simulink model "Laser_Knight_Team9"  (R2019a)
settings: Solver=VariableStepAuto  StartTime=0.0  StopTime=10.0  RelTol=1e-3
libraries: arduinolib x34
settings Model: Creator=user  LastModifiedBy=user

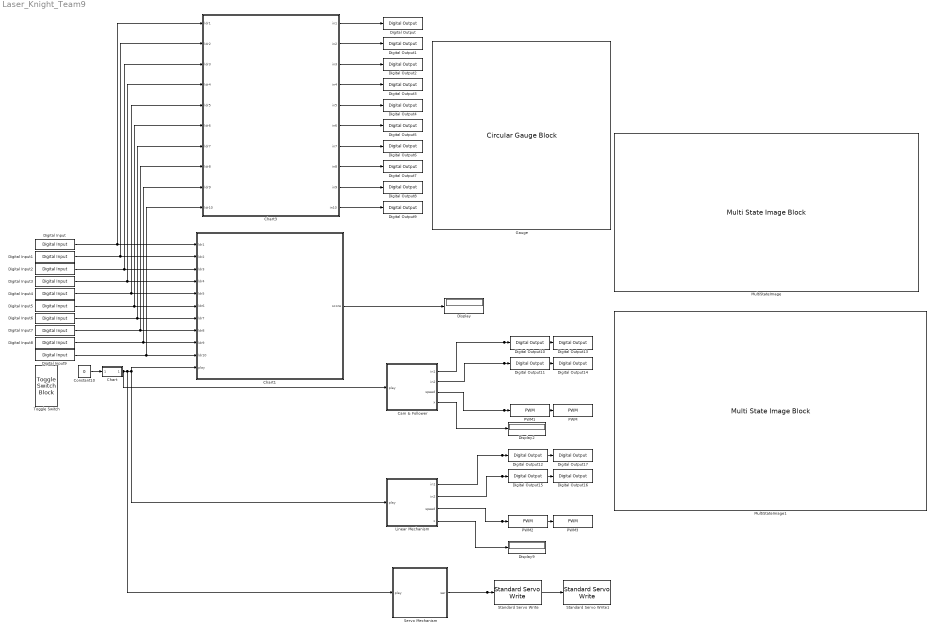
== system Laser_Knight_Team9 ==
  Cam & Follower : Stateflow chart  BlockKeywords=__PRM__SERIALIZED__DATA__:Stateflow Chart,Stateflow Diagram  TreatAsAtomicUnit=on
  Chart : Stateflow chart  BlockKeywords=__PRM__SERIALIZED__DATA__:Stateflow Chart,Stateflow Diagram  TreatAsAtomicUnit=on
  Chart1 : Stateflow chart  BlockKeywords=__PRM__SERIALIZED__DATA__:Stateflow Chart,Stateflow Diagram  TreatAsAtomicUnit=on
  Chart3 : Stateflow chart  BlockKeywords=__PRM__SERIALIZED__DATA__:Stateflow Chart,Stateflow Diagram  TreatAsAtomicUnit=on
  Constant10 : Constant  Value=0
  Digital Input : arduinolib/Digital Input  pinNumber=22  sampleTime=0.001  blockPlatform=arduino
      settings: SourceProductName=Simulink Support Package for Arduino Hardware
  Digital Input1 : arduinolib/Digital Input  pinNumber=24  sampleTime=0.1  blockPlatform=arduino
      settings: SourceProductName=Simulink Support Package for Arduino Hardware
  Digital Input2 : arduinolib/Digital Input  pinNumber=26  sampleTime=0.1  blockPlatform=arduino
      settings: SourceProductName=Simulink Support Package for Arduino Hardware
  Digital Input3 : arduinolib/Digital Input  pinNumber=28  sampleTime=0.1  blockPlatform=arduino
      settings: SourceProductName=Simulink Support Package for Arduino Hardware
  Digital Input4 : arduinolib/Digital Input  pinNumber=30  sampleTime=0.1  blockPlatform=arduino
      settings: SourceProductName=Simulink Support Package for Arduino Hardware
  Digital Input5 : arduinolib/Digital Input  pinNumber=32  sampleTime=0.1  blockPlatform=arduino
      settings: SourceProductName=Simulink Support Package for Arduino Hardware
  Digital Input6 : arduinolib/Digital Input  pinNumber=34  sampleTime=0.1  blockPlatform=arduino
      settings: SourceProductName=Simulink Support Package for Arduino Hardware
  Digital Input7 : arduinolib/Digital Input  pinNumber=36  sampleTime=0.1  blockPlatform=arduino
      settings: SourceProductName=Simulink Support Package for Arduino Hardware
  Digital Input8 : arduinolib/Digital Input  pinNumber=38  sampleTime=0.1  blockPlatform=arduino
      settings: SourceProductName=Simulink Support Package for Arduino Hardware
  Digital Input9 : arduinolib/Digital Input  pinNumber=40  sampleTime=0.1  blockPlatform=arduino
      settings: SourceProductName=Simulink Support Package for Arduino Hardware
  Digital Output : arduinolib/Digital Output  pinNumber=42  blockPlatform=arduino
  Digital Output1 : arduinolib/Digital Output  pinNumber=44  blockPlatform=arduino
  Digital Output10 : arduinolib/Digital Output  pinNumber=8  blockPlatform=arduino
  Digital Output11 : arduinolib/Digital Output  pinNumber=10  blockPlatform=arduino
  Digital Output12 : arduinolib/Digital Output  pinNumber=12  blockPlatform=arduino
  Digital Output13 : arduinolib/Digital Output  pinNumber=9  blockPlatform=arduino
  Digital Output14 : arduinolib/Digital Output  pinNumber=11  blockPlatform=arduino
  Digital Output15 : arduinolib/Digital Output  pinNumber=14  blockPlatform=arduino
  Digital Output16 : arduinolib/Digital Output  pinNumber=15  blockPlatform=arduino
  Digital Output17 : arduinolib/Digital Output  pinNumber=13  blockPlatform=arduino
  Digital Output2 : arduinolib/Digital Output  pinNumber=46  blockPlatform=arduino
  Digital Output3 : arduinolib/Digital Output  pinNumber=48  blockPlatform=arduino
  Digital Output4 : arduinolib/Digital Output  pinNumber=50  blockPlatform=arduino
  Digital Output5 : arduinolib/Digital Output  pinNumber=52  blockPlatform=arduino
  Digital Output6 : arduinolib/Digital Output  pinNumber=37  blockPlatform=arduino
  Digital Output7 : arduinolib/Digital Output  pinNumber=39  blockPlatform=arduino
  Digital Output8 : arduinolib/Digital Output  pinNumber=41  blockPlatform=arduino
  Digital Output9 : arduinolib/Digital Output  pinNumber=43  blockPlatform=arduino
  Display : Display
  Display2 : Display
  Display9 : Display
  Gauge : CircularGaugeBlock  LabelPosition=Hide  ScaleMax=300  TickInterval=20
  Linear Mechanism : Stateflow chart  BlockKeywords=__PRM__SERIALIZED__DATA__:Stateflow Chart,Stateflow Diagram  TreatAsAtomicUnit=on
  MultiStateImage : MultiStateImageBlock  LabelPosition=Hide  ScaleMode=Fill
  MultiStateImage1 : MultiStateImageBlock  LabelPosition=Hide  ScaleMode=Fill
  PWM : arduinolib/PWM  pinNumber=4  EnableInputFrequency=off  InitialFrequency=2000  InitialDutyCycle=0  NotificationType=None  blockPlatform=arduino
  PWM1 : arduinolib/PWM  pinNumber=5  EnableInputFrequency=off  InitialFrequency=2000  InitialDutyCycle=0  NotificationType=None  blockPlatform=arduino
  PWM2 : arduinolib/PWM  pinNumber=6  EnableInputFrequency=off  InitialFrequency=2000  InitialDutyCycle=0  NotificationType=None  blockPlatform=arduino
  PWM3 : arduinolib/PWM  pinNumber=7  EnableInputFrequency=off  InitialFrequency=2000  InitialDutyCycle=0  NotificationType=None  blockPlatform=arduino
  Servo Mechanism : Stateflow chart  BlockKeywords=__PRM__SERIALIZED__DATA__:Stateflow Chart,Stateflow Diagram  TreatAsAtomicUnit=on
  Standard Servo Write : arduinolib/Standard Servo Write  pinNumber=31  ServoIndex=0  blockPlatform=ARDUINO
      settings: SourceProductName=Simulink Support Package for Arduino Hardware
  Standard Servo Write1 : arduinolib/Standard Servo Write  pinNumber=33  ServoIndex=0  blockPlatform=ARDUINO
      settings: SourceProductName=Simulink Support Package for Arduino Hardware
  Toggle Switch : ToggleSwitchBlock  LabelPosition=Hide
      settings: Values={{'Off', 'On'}, [0 1]}
  wires:
  Chart3/5(in5) -> Digital Output4/1
  Linear Mechanism/4(x) -> Display9/1
  Chart3/8(in8) -> Digital Output7/1
  Servo Mechanism/1(ser) -> Standard Servo Write1/1, Standard Servo Write/1
  Chart3/3(in3) -> Digital Output2/1
  Cam & Follower/4(x) -> Display2/1
  Cam & Follower/1(in1) -> Digital Output13/1, Digital Output10/1
  Cam & Follower/3(speed) -> PWM/1, PWM1/1
  Cam & Follower/2(in2) -> Digital Output14/1, Digital Output11/1
  Digital Input6/1 -> Chart3/7(ldr7), Chart1/7(ldr7)
  Digital Input4/1 -> Chart3/5(ldr5), Chart1/5(ldr5)
  Digital Input2/1 -> Chart3/3(ldr3), Chart1/3(ldr3)
  Digital Input5/1 -> Chart3/6(ldr6), Chart1/6(ldr6)
  Digital Input/1 -> Chart3/1(ldr1), Chart1/1(ldr1)
  Digital Input7/1 -> Chart3/8(ldr8), Chart1/8(ldr8)
  Linear Mechanism/3(speed) -> PWM3/1, PWM2/1
  Digital Input9/1 -> Chart3/10(ldr10), Chart1/10(ldr10)
  Digital Input8/1 -> Chart3/9(ldr9), Chart1/9(ldr9)
  Chart/1(play) -> Cam & Follower/1(play), Servo Mechanism/1(play), Linear Mechanism/1(play), Chart1/11(play)
  Linear Mechanism/2(in2) -> Digital Output16/1, Digital Output15/1
  Digital Input3/1 -> Chart3/4(ldr4), Chart1/4(ldr4)
  Chart3/4(in4) -> Digital Output3/1
  Chart3/1(in1) -> Digital Output/1
  Chart1/1(score) -> Display/1
  Digital Input1/1 -> Chart3/2(ldr2), Chart1/2(ldr2)
  Chart3/10(in10) -> Digital Output9/1
  Chart3/2(in2) -> Digital Output1/1
  Chart3/6(in6) -> Digital Output5/1
  Chart3/7(in7) -> Digital Output6/1
  Constant10/1 -> Chart/1(game)
  Chart3/9(in9) -> Digital Output8/1
  Linear Mechanism/1(in1) -> Digital Output17/1, Digital Output12/1

== stateflow chart Laser_Knight_Team9/Chart1 ==
  state Gameplay
    state initial
      score=0;
    state Score
      state LDR1 [parallel]
        settings: executionOrder=1
        state Score1
          score=score;
        state LDR1
          score=score;
        (default) -> Gameplay.Score.LDR1.Score1
        Gameplay.Score.LDR1.Score1 -> Gameplay.Score.LDR1.LDR1 : [ldr1==0||ldr2==0]{score=score+10;}
        Gameplay.Score.LDR1.LDR1 -> Gameplay.Score.LDR1.Score1 : [after(3,sec)]
      state LDR2 [parallel]
        settings: executionOrder=2
        state Score1
          score=score;
        state LDR1
          score=score;
        (default) -> Gameplay.Score.LDR2.Score1
        Gameplay.Score.LDR2.Score1 -> Gameplay.Score.LDR2.LDR1 : [ldr3==0||ldr4==0]{score=score+20}
        Gameplay.Score.LDR2.LDR1 -> Gameplay.Score.LDR2.Score1 : [after(3,sec)]
      state LDR3 [parallel]
        settings: executionOrder=3
        state Score1
          score=score;
        state LDR1
          score=score;
        (default) -> Gameplay.Score.LDR3.Score1
        Gameplay.Score.LDR3.Score1 -> Gameplay.Score.LDR3.LDR1 : [ldr5==0||ldr6==0]{score=score+30}
        Gameplay.Score.LDR3.LDR1 -> Gameplay.Score.LDR3.Score1 : [after(3,sec)]
      state LDR4 [parallel]
        settings: executionOrder=4
        state Score1
          score=score;
        state LDR1
          score=score;
        (default) -> Gameplay.Score.LDR4.Score1
        Gameplay.Score.LDR4.Score1 -> Gameplay.Score.LDR4.LDR1 : [ldr7==0||ldr8==0]{score=score+40}
        Gameplay.Score.LDR4.LDR1 -> Gameplay.Score.LDR4.Score1 : [after(3,sec)]
      state LDR5 [parallel]
        settings: executionOrder=5
        state Score1
          score=score;
        state LDR1
          score=score;
        (default) -> Gameplay.Score.LDR5.Score1
        Gameplay.Score.LDR5.Score1 -> Gameplay.Score.LDR5.LDR1 : [ldr9==0||ldr10==0]{score=score+50}
        Gameplay.Score.LDR5.LDR1 -> Gameplay.Score.LDR5.Score1 : [after(3,sec)]
    (default) -> initial
    initial -> Score
  state GameOver
    score=score;
  (default) -> Gameplay
  Gameplay -> GameOver : [play==0]
  GameOver -> Gameplay : [play==1]
  data: score output; ldr1 input; ldr2 input; ldr3 input; ldr4 input; ldr5 input; ldr6 input; ldr7 input; ldr8 input; ldr9 input; ldr10 input; play input

== stateflow chart Laser_Knight_Team9/Servo Mechanism ==
  state move1
    ser=ser;
  state initial
    ser=10
  state move2
    ser=ser;
  move1 -> move1 [order 2] : [after(50,msec)&&ser<170]{ser = ser + 1}
  (default) -> initial
  initial -> move1 : [play==1]
  move1 -> move2 [order 1] : [ser==170]
  move2 -> move1 [order 1] : [ser==10]
  move2 -> initial [order 3] : [play==0]
  move2 -> move2 [order 2] : [after(50,msec)&&ser>10]{ser = ser - 1}
  data: ser output; play input

== stateflow chart Laser_Knight_Team9/Cam & Follower ==
  state Gameplay
    x=2;
    state Initial
      speed=200;
      in1=0;
      in2=0;
    state Final
      state Motor2
        speed=speed
        in1=1
        in2=0
        x=0
      state Motor1
        speed=speed
        in1=0
        in2=1
        x=0
      (default) -> Motor1
      Motor2 -> Motor1 : [after(10,sec)]{speed=speed+5}
      Motor1 -> Motor2 : [after(10,sec)]{speed=speed+5}
    (default) -> Initial
    Initial -> Final : [speed==200 && play==1]
    Final -> Initial : [speed>=255]
  state GameOver
    x=1;
    in1=0;
    in2=0;
    speed=200;
  (default) -> Gameplay
  Gameplay -> GameOver : [play==0]
  GameOver -> Gameplay : [x==1&&play==1]
  data: in1 output; in2 output; speed output; x output =0; play input

== stateflow chart Laser_Knight_Team9/Chart ==
  state Time
    t=180;
    state Time1
      t=t;
      play=1;
    state Time2
      t=t;
      play=1;
    Time1 -> Time2 : [after(1,sec)&&game==1]{t = t - 1}
    (default) -> Time1
    Time2 -> Time1 : [after(1,sec)&&game==1]{t = t - 1}
  state GameOver
    play=0;
  (default) -> Time
  Time -> GameOver : [t==0 || game==0]
  GameOver -> Time : [game==1]
  data: play output =1; t local =180; game input

== stateflow chart Laser_Knight_Team9/Linear Mechanism ==
  state Gameplay
    state Final
      state Motor2
        speed=255
        in1=1
        in2=0
        x=0
      state Motor1
        speed=255
        in1=0
        in2=1
        x=0
      (default) -> Motor1
      Motor2 -> Motor1 : [after(8,sec)&&play==1]
      Motor1 -> Motor2 : [after(8,sec)&&play==1]
  state GameOver
    x=1;
    in1=0;
    in2=0;
    speed=200;
  (default) -> Gameplay
  Gameplay -> GameOver : [play==0]
  GameOver -> Gameplay : [play==1&&x==1]
  data: in1 output; in2 output; speed output; x output; play input

== stateflow chart Laser_Knight_Team9/Chart3 ==
  state LEDs
    state LDR1 [parallel]
      settings: executionOrder=1
      state On
        in1=1;
      state Off
        in1=0;
      state Off1
        in1=0;
      (default) -> LEDs.LDR1.On
      LEDs.LDR1.On -> LEDs.LDR1.Off : [ldr1==0]
      LEDs.LDR1.Off1 -> LEDs.LDR1.On : [after(3,sec)]
      LEDs.LDR1.Off -> LEDs.LDR1.Off1 : [ldr1==1]
    state LDR2 [parallel]
      settings: executionOrder=2
      state On
        in2=1;
      state Off
        in2=0;
      state Off1
        in2=0;
      (default) -> LEDs.LDR2.On
      LEDs.LDR2.On -> LEDs.LDR2.Off : [ldr2==0]
      LEDs.LDR2.Off1 -> LEDs.LDR2.On : [after(3,sec)]
      LEDs.LDR2.Off -> LEDs.LDR2.Off1 : [ldr2==1]
    state LDR3 [parallel]
      settings: executionOrder=3
      state On
        in3=1;
      state Off
        in3=0;
      state Off1
        in3=0;
      (default) -> LEDs.LDR3.On
      LEDs.LDR3.On -> LEDs.LDR3.Off : [ldr3==0]
      LEDs.LDR3.Off1 -> LEDs.LDR3.On : [after(3,sec)]
      LEDs.LDR3.Off -> LEDs.LDR3.Off1 : [ldr3==1]
    state LDR4 [parallel]
      settings: executionOrder=4
      state On
        in4=1;
      state Off
        in4=0;
      state Off1
        in1=0;
      (default) -> LEDs.LDR4.On
      LEDs.LDR4.On -> LEDs.LDR4.Off : [ldr4==0]
      LEDs.LDR4.Off1 -> LEDs.LDR4.On : [after(3,sec)]
      LEDs.LDR4.Off -> LEDs.LDR4.Off1 : [ldr4==1]
    state LDR5 [parallel]
      settings: executionOrder=5
      state On
        in5=1;
      state Off
        in5=0;
      state Off1
        in5=0;
      (default) -> LEDs.LDR5.On
      LEDs.LDR5.On -> LEDs.LDR5.Off : [ldr5==0]
      LEDs.LDR5.Off1 -> LEDs.LDR5.On : [after(3,sec)]
      LEDs.LDR5.Off -> LEDs.LDR5.Off1 : [ldr5==1]
    state LDR6 [parallel]
      settings: executionOrder=6
      state On
        in6=1;
      state Off
        in6=0;
      state Off1
        in6=0;
      (default) -> LEDs.LDR6.On
      LEDs.LDR6.On -> LEDs.LDR6.Off : [ldr6==0]
      LEDs.LDR6.Off1 -> LEDs.LDR6.On : [after(3,sec)]
      LEDs.LDR6.Off -> LEDs.LDR6.Off1 : [ldr6==1]
    state LDR7 [parallel]
      settings: executionOrder=7
      state On
        in7=1;
      state Off
        in7=0;
      state Off1
        in7=0;
      (default) -> LEDs.LDR7.On
      LEDs.LDR7.On -> LEDs.LDR7.Off : [ldr7==0]
      LEDs.LDR7.Off1 -> LEDs.LDR7.On : [after(3,sec)]
      LEDs.LDR7.Off -> LEDs.LDR7.Off1 : [ldr7==1]
    state LDR8 [parallel]
      settings: executionOrder=8
      state On
        in8=1;
      state Off
        in8=0;
      state Off1
        in8=0;
      (default) -> LEDs.LDR8.On
      LEDs.LDR8.On -> LEDs.LDR8.Off : [ldr8==0]
      LEDs.LDR8.Off1 -> LEDs.LDR8.On : [after(3,sec)]
      LEDs.LDR8.Off -> LEDs.LDR8.Off1 : [ldr8==1]
    state LDR9 [parallel]
      settings: executionOrder=9
      state On
        in9=1;
      state Off
        in9=0;
      state Off1
        in9=0;
      (default) -> LEDs.LDR9.On
      LEDs.LDR9.On -> LEDs.LDR9.Off : [ldr9==0]
      LEDs.LDR9.Off1 -> LEDs.LDR9.On : [after(3,sec)]
      LEDs.LDR9.Off -> LEDs.LDR9.Off1 : [ldr9==1]
    state LDR10 [parallel]
      settings: executionOrder=10
      state On
        in10=1;
      state Off
        in10=0;
      state Off1
        in10=0;
      (default) -> LEDs.LDR10.On
      LEDs.LDR10.On -> LEDs.LDR10.Off : [ldr10==0]
      LEDs.LDR10.Off1 -> LEDs.LDR10.On : [after(3,sec)]
      LEDs.LDR10.Off -> LEDs.LDR10.Off1 : [ldr10==1]
  (default) -> LEDs
  data: ldr1 input; in1 output; ldr2 input; ldr3 input; ldr4 input; ldr5 input; ldr6 input; ldr7 input; ldr8 input; ldr9 input; ldr10 input; in2 output; in3 output; in4 output; in5 output; in6 output; in7 output; in8 output; in9 output; in10 output
